simulink model "system"  (R2024b)
settings: Solver=VariableStepAuto  StartTime=0.0  StopTime=10.0  RelTol=1e-3
settings Model: Creator=SEBAS  LastModifiedBy=SEBAS
settings DataIOCC: ReturnWorkspaceOutputs=off

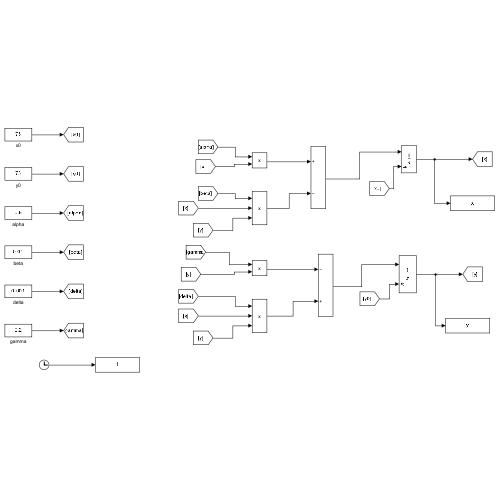
[thumbnail: Simulink's stored preview of the top-level diagram]
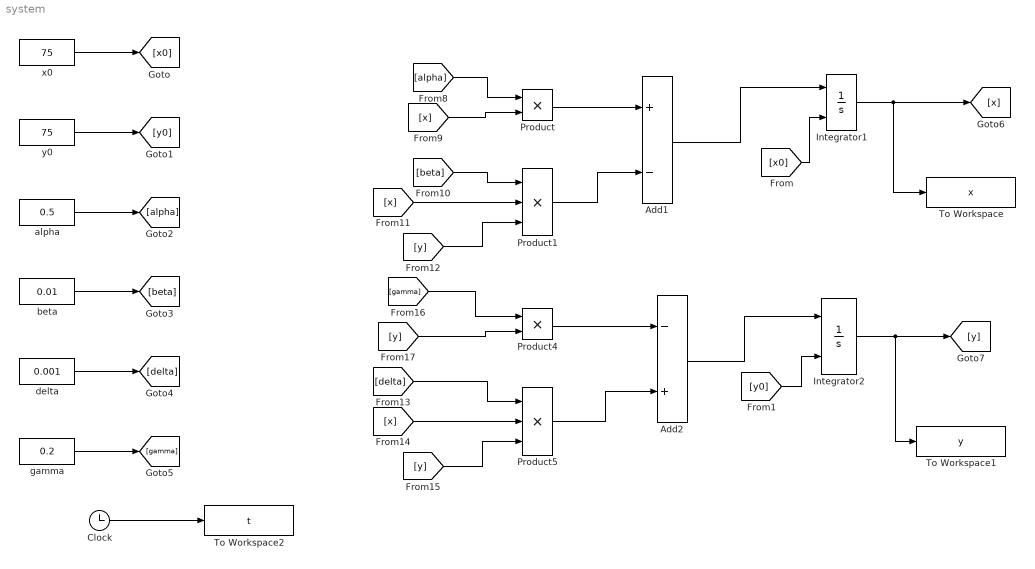
== system system ==
  Add1 : Sum  Inputs=+-
  Add2 : Sum  Inputs=-+
  Clock : Clock
  Integrator1 : Integrator  InitialConditionSource=external
  Integrator2 : Integrator  InitialConditionSource=external
  Product : Product
  Product1 : Product  Inputs=3
  Product4 : Product
  Product5 : Product  Inputs=3
  To Workspace : ToWorkspace  VariableName=x  SampleTime=-1
  To Workspace1 : ToWorkspace  VariableName=y  SampleTime=-1
  To Workspace2 : ToWorkspace  VariableName=t  SampleTime=-1
  alpha : Constant  Value=0.5
  beta : Constant  Value=0.01
  delta : Constant  Value=0.001
  gamma : Constant  Value=0.2
  x0 : Constant  Value=75
  y0 : Constant  Value=75
  wires:
  x0/1 -> [x0]
  y0/1 -> [y0]
  alpha/1 -> [alpha]
  beta/1 -> [beta]
  delta/1 -> [delta]
  gamma/1 -> [gamma]
  Integrator2/1 -> To Workspace1/1, [y]
  Integrator1/1 -> To Workspace/1, [x]
  Product/1 -> Add1/1
  Product1/1 -> Add1/2
  [alpha] -> Product/1
  [x] -> Product/2
  [beta] -> Product1/1
  [x] -> Product1/2
  [y] -> Product1/3
  [delta] -> Product5/1
  [y] -> Product5/3
  [x] -> Product5/2
  [y] -> Product4/2
  [gamma] -> Product4/1
  Product5/1 -> Add2/2
  Product4/1 -> Add2/1
  [x0] -> Integrator1/2
  [y0] -> Integrator2/2
  Add2/1 -> Integrator2/1
  Add1/1 -> Integrator1/1
  Clock/1 -> To Workspace2/1
